simulink model "FlSys_FlCons"  (R2016b)
settings: configuration reference "CodeGenConfigSet" (kept outside this file)
values from neighbouring files (symbols this model uses):
  Epm_numCyl_C = Calibration.Parameter    [init_FlSys_FlCons.m]
undefined symbols (not defined in the file or in its folder): Switch_conv
settings Model: Creator=Administrator  LastModifiedBy=Administrator
settings ConfigSetRef: SourceLocation=Base Workspace

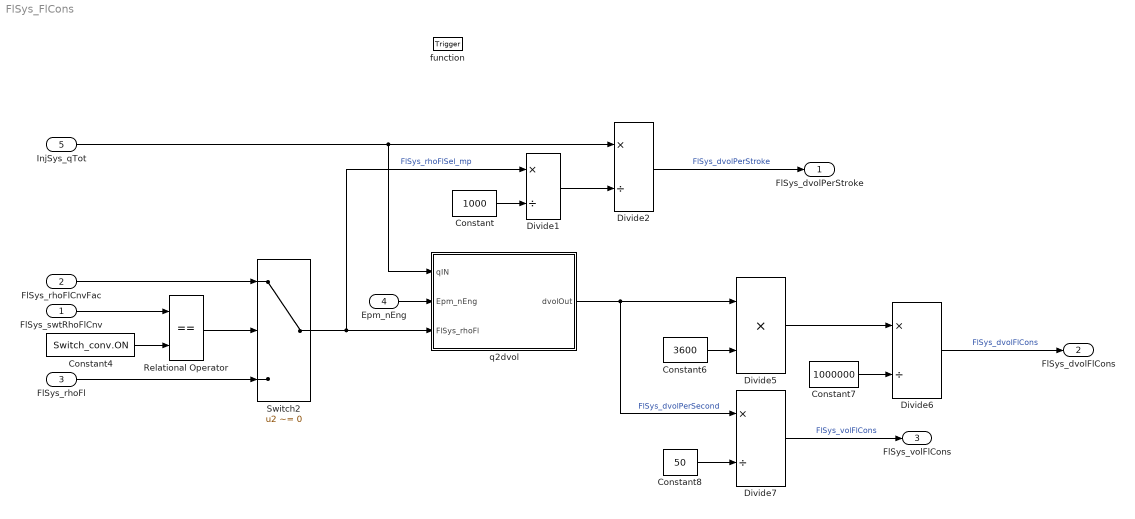
== system FlSys_FlCons ==
  FlSys_swtRhoFlCnv : Inport  Description=switch for customer specific fuel conversion factor  OutDataTypeStr=Enum: Switch_conv
  FlSys_rhoFlCnvFac : Inport  Tag=kg/m^3  Description=customer specific fuel conversion factor  Port=2  OutMin=0  OutMax=3276  OutDataTypeStr=Fuel_Rho_kg_m3
  FlSys_rhoFl : Inport  Tag=kg/m^3  Description=Fuel density coefficient  Port=3  OutMin=0  OutMax=3276  OutDataTypeStr=Fuel_Rho_kg_m3
  Epm_nEng : Inport  Tag=rpm  Description=Engine speed  Port=4  OutMin=0  OutMax=6000  OutDataTypeStr=EngSpeed_rpm
  InjSys_qTot : Inport  Tag=mg/hub  Description=Total engine injection quantity  Port=5  OutMin=-319  OutMax=319  OutDataTypeStr=FuelMass_mg_hub
  function : TriggerPort  TriggerType=function-call  VariantControl=Variant
  Constant : Constant  Value=1000  OutDataTypeStr=uint16
  Constant4 : Constant  Value=Switch_conv.ON
  Constant6 : Constant  Value=3600  OutDataTypeStr=uint16
  Constant7 : Constant  Value=1000000  OutDataTypeStr=int32
  Constant8 : Constant  Value=50  OutDataTypeStr=int16
  Divide1 : Product  Inputs=*/  OutDataTypeStr=fixdt(1,16,7)  SaturateOnIntegerOverflow=on
  Divide2 : Product  Inputs=*/  OutDataTypeStr=Inherit: Inherit via back propagation  SaturateOnIntegerOverflow=on
  Divide5 : Product  Inputs=**  OutDataTypeStr=fixdt(1,32,5)  SaturateOnIntegerOverflow=on
  Divide6 : Product  Inputs=*/  OutDataTypeStr=Inherit: Inherit via back propagation  SaturateOnIntegerOverflow=on
  Divide7 : Product  Inputs=*/  OutDataTypeStr=Inherit: Inherit via back propagation  SaturateOnIntegerOverflow=on
  Relational Operator : RelationalOperator  Operator===  OutDataTypeStr=boolean  RndMeth=Simplest  InputSameDT=on
  Switch2 : Switch  Criteria=u2 ~= 0  SaturateOnIntegerOverflow=on  InputSameDT=on
  q2dvol : Subsystem
  FlSys_dvolPerStroke : Outport  Tag=mm^3/hub  Description=fuel volumina per stroke ul/stroke  OutMin=0  OutMax=3276  OutDataTypeStr=FuelMass_mm3_hub
  FlSys_dvolFlCons : Outport  Tag=L/h  Description=Fuel consumption [l/h]  Port=2  OutMin=0  OutMax=327  OutDataTypeStr=FlCon_L_h
  FlSys_volFlCons : Outport  Tag=ul/20ms  Description=absolute fuel consumption in ul/DT  Port=3  OutMin=-2147483648  OutMax=2147483647  OutDataTypeStr=FlConsum_ul_20ms
  wires:
  InjSys_qTot/1 -> Divide2/1, q2dvol/1(qIN)
  FlSys_swtRhoFlCnv/1 -> Relational Operator/1
  FlSys_rhoFlCnvFac/1 -> Switch2/1
  FlSys_rhoFl/1 -> Switch2/3
  Switch2/1 -> Divide1/1, q2dvol/3(FlSys_rhoFl)  "FlSys_rhoFlSel_mp"
  Constant4/1 -> Relational Operator/2
  Relational Operator/1 -> Switch2/2
  q2dvol/1(dvolOut) -> Divide5/1, Divide7/1  "FlSys_dvolPerSecond"
  Constant6/1 -> Divide5/2
  Divide5/1 -> Divide6/1
  Constant7/1 -> Divide6/2
  Divide6/1 -> FlSys_dvolFlCons/1  "FlSys_dvolFlCons"
  Constant8/1 -> Divide7/2
  Divide7/1 -> FlSys_volFlCons/1  "FlSys_volFlCons"
  Divide2/1 -> FlSys_dvolPerStroke/1  "FlSys_dvolPerStroke"
  Epm_nEng/1 -> q2dvol/2(Epm_nEng)
  Divide1/1 -> Divide2/2
  Constant/1 -> Divide1/2

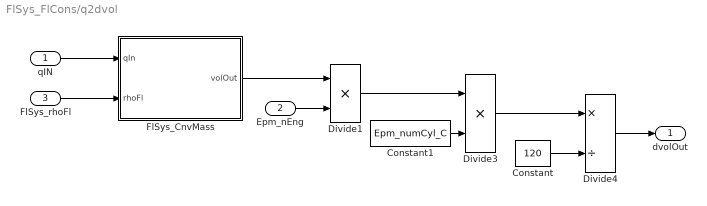
== system FlSys_FlCons/q2dvol ==
  qIN : Inport
  Epm_nEng : Inport  Port=2
  FlSys_rhoFl : Inport  Port=3
  Constant : Constant  Value=120  OutDataTypeStr=uint16
  Constant1 : Constant  Description=Cylinder number  Value=Epm_numCyl_C
  Divide1 : Product  Inputs=**  OutDataTypeStr=fixdt(1,32,5)  SaturateOnIntegerOverflow=on
  Divide3 : Product  Inputs=**  OutDataTypeStr=fixdt(1,32,5)  SaturateOnIntegerOverflow=on
  Divide4 : Product  Inputs=*/  OutDataTypeStr=Inherit: Inherit via back propagation  SaturateOnIntegerOverflow=on
  FlSys_CnvMass : Subsystem
  dvolOut : Outport
  wires:
  FlSys_rhoFl/1 -> FlSys_CnvMass/2(rhoFl)
  qIN/1 -> FlSys_CnvMass/1(qIn)
  Divide4/1 -> dvolOut/1
  FlSys_CnvMass/1(volOut) -> Divide1/1
  Constant/1 -> Divide4/2
  Epm_nEng/1 -> Divide1/2
  Constant1/1 -> Divide3/2
  Divide1/1 -> Divide3/1
  Divide3/1 -> Divide4/1

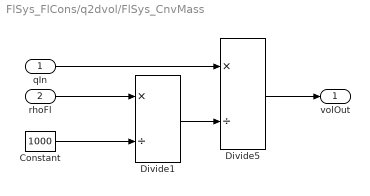
== system FlSys_FlCons/q2dvol/FlSys_CnvMass ==
  qIn : Inport
  rhoFl : Inport  Port=2
  Constant : Constant  Value=1000  OutDataTypeStr=uint16
  Divide1 : Product  Inputs=*/  OutDataTypeStr=fixdt(1,16,7)  SaturateOnIntegerOverflow=on
  Divide5 : Product  Inputs=*/  OutDataTypeStr=FuelMass_mm3_hub  SaturateOnIntegerOverflow=on
  volOut : Outport
  wires:
  Divide5/1 -> volOut/1
  rhoFl/1 -> Divide1/1
  qIn/1 -> Divide5/1
  Constant/1 -> Divide1/2
  Divide1/1 -> Divide5/2
